simulink model "Actuator_model_discrete"  (R2015b)
settings: Solver=FixedStepAuto  StartTime=0.0  StopTime=50  FixedStep=0.004  RelTol=1e-3
values from neighbouring files (symbols this model uses):
  Bv = 10 / ((180/pi) * 1000)    (= 0.000174532925199)    [initialize_param_mdeg.m]    (also in intialize_param.m = 8)
  Jeq = 0.2740    (= 0.274)    [initialize_param_mdeg.m]    (also in intialize_param.m)
  Km = 0.0429    [initialize_param_mdeg.m]    (also in intialize_param.m)
  Kp = wn / (2*zeta)    (= 4297183.46348)    [initialize_param_mdeg.m]    (also in intialize_param.m = 50)
  Kr = 160    [initialize_param_mdeg.m]    (also in intialize_param.m)
  Kv = wn^2 * Bv / (Kp*Kr*Km)    (= 437.062937063)    [initialize_param_mdeg.m]    (also in intialize_param.m = 233.1002331)
  Tv = (Jeq/Bv)    (= 1569.90435866)    [initialize_param_mdeg.m]    (also in intialize_param.m = 0.03425)
settings Model: Creator=mohit  LastModifiedBy=mohit
settings SolverCC: ZeroCrossControl=DisableAll

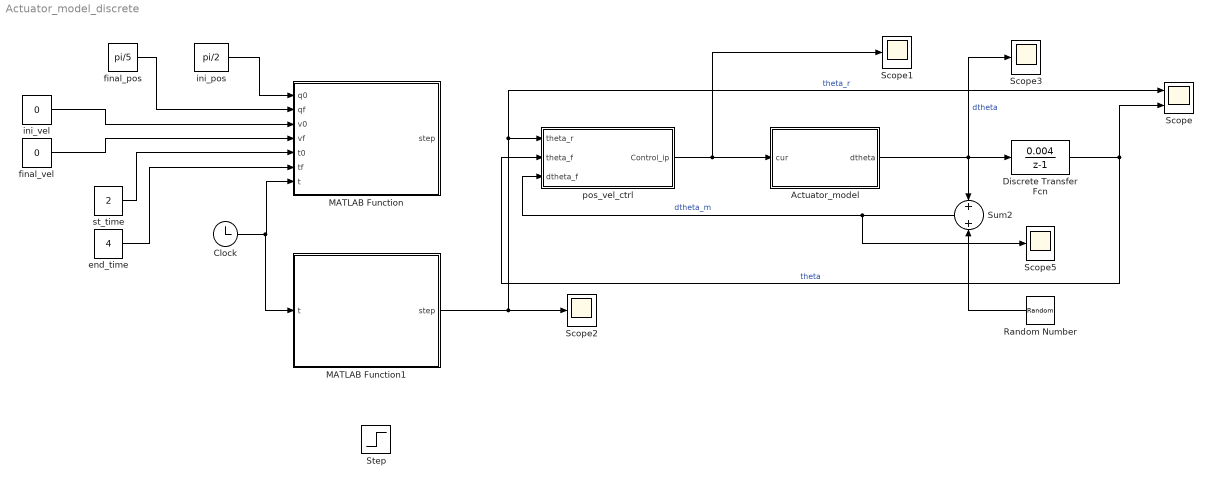
== system Actuator_model_discrete ==
  Actuator_model : Subsystem
  Clock : Clock
  Discrete Transfer Fcn : DiscreteTransferFcn  Numerator=[0.004]  Denominator=[1 -1]
  MATLAB Function : MATLAB Function  TreatAsAtomicUnit=on
  MATLAB Function1 : MATLAB Function  TreatAsAtomicUnit=on
  Random Number : RandomNumber  Variance=0.001 * (pi / 180) * 1000  SampleTime=0.004
  Scope : Scope  NumInputPorts=2
  Scope{1..3,5} (4 alike) : Scope
  Step : Step  Time=4  After=pi/2  SampleTime=0.004
  Sum2 : Sum
  end_time : Constant  Value=4
  final_pos : Constant  Value=pi/5
  final_vel : Constant  Value=0
  ini_pos : Constant  Value=pi/2
  ini_vel : Constant  Value=0
  pos_vel_ctrl : Subsystem
  st_time : Constant  Value=2
  wires:
  Discrete Transfer Fcn/1 -> Scope/2, pos_vel_ctrl/2(theta_f)  "theta"
  Actuator_model/1(dtheta) -> Scope3/1, Discrete Transfer Fcn/1, Sum2/1  "dtheta"
  Sum2/1 -> pos_vel_ctrl/3(dtheta_f), Scope5/1  "dtheta_m"
  Clock/1 -> MATLAB Function1/1(t), MATLAB Function/7(t)
  ini_pos/1 -> MATLAB Function/1(q0)
  final_pos/1 -> MATLAB Function/2(qf)
  ini_vel/1 -> MATLAB Function/3(v0)
  final_vel/1 -> MATLAB Function/4(vf)
  st_time/1 -> MATLAB Function/5(t0)
  end_time/1 -> MATLAB Function/6(tf)
  Random Number/1 -> Sum2/2
  pos_vel_ctrl/1(Control_ip) -> Scope1/1, Actuator_model/1(cur)
  MATLAB Function1/1(step) -> Scope/1, pos_vel_ctrl/1(theta_r), Scope2/1  "theta_r"

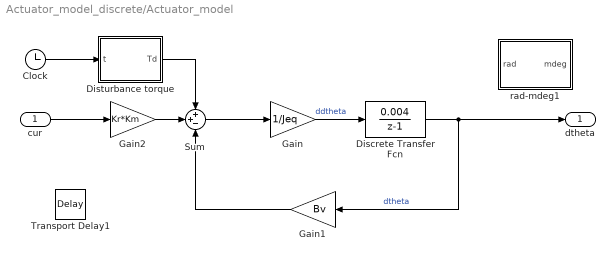
== system Actuator_model_discrete/Actuator_model ==
  cur : Inport
  Clock : Clock
  Discrete Transfer Fcn : DiscreteTransferFcn  Numerator=[0.004]  Denominator=[1 -1]
  Disturbance torque : MATLAB Function  TreatAsAtomicUnit=on
  Gain : Gain  Gain=1/Jeq
  Gain1 : Gain  Gain=Bv
  Gain2 : Gain  Gain=Kr*Km
  Sum : Sum  Inputs=++-
  Transport Delay1 : TransportDelay  DelayTime=0.004
  rad-mdeg1 : MATLAB Function  TreatAsAtomicUnit=on
  dtheta : Outport
  wires:
  Gain2/1 -> Sum/2
  Sum/1 -> Gain/1
  Gain1/1 -> Sum/3
  Gain/1 -> Discrete Transfer Fcn/1  "ddtheta"
  Clock/1 -> Disturbance torque/1(t)
  Disturbance torque/1(Td) -> Sum/1
  cur/1 -> Gain2/1
  Discrete Transfer Fcn/1 -> dtheta/1, Gain1/1  "dtheta"

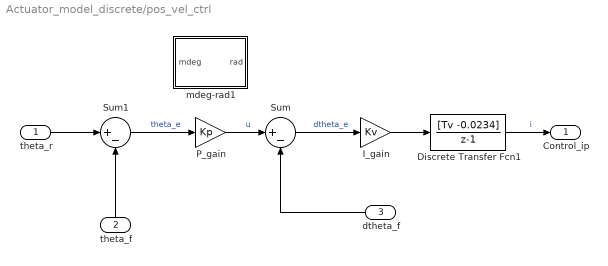
== system Actuator_model_discrete/pos_vel_ctrl ==
  theta_r : Inport
  theta_f : Inport  Port=2
  dtheta_f : Inport  Port=3
  Discrete Transfer Fcn1 : DiscreteTransferFcn  Numerator=[Tv -0.0234]  Denominator=[1 -1]
  I_gain : Gain  Gain=Kv
  P_gain : Gain  Gain=Kp
  Sum : Sum  Inputs=|+-
  Sum1 : Sum  Inputs=|+-
  mdeg-rad1 : MATLAB Function  TreatAsAtomicUnit=on
  Control_ip : Outport
  wires:
  theta_r/1 -> Sum1/1
  dtheta_f/1 -> Sum/2
  theta_f/1 -> Sum1/2
  Discrete Transfer Fcn1/1 -> Control_ip/1  "i"
  Sum/1 -> I_gain/1  "dtheta_e"
  Sum1/1 -> P_gain/1  "theta_e"
  P_gain/1 -> Sum/1  "u"
  I_gain/1 -> Discrete Transfer Fcn1/1

== matlab function Actuator_model_discrete/MATLAB Function ==
  settings: updateMethod=DISCRETE  sampleTime=0.004
  data: q0 input; qf input; v0 input; vf input; t0 input; tf input; t input; step output
function step = smoothstep(q0,qf,v0,vf,t0,tf,t)
    Q = [q0 v0 qf vf]';
    T = zeros(4); A = zeros(4,1);
    ti = 0;
    tn = tf-t0;
    T = [1 ti ti^2  ti^3; ...
         0  1  2*ti 3*ti^2; ...
         1 tn tn^2  tn^3; ...
         0  1  2*tn 3*tn^2];
    A = T \ Q;

    if t <= t0
        step = q0;

    elseif t > t0 && t <= tf
        step = A(4)*((t-t0)^3) + A(3)*((t-t0)^2) + A(2)*(t-t0) + A(1);
    
    else
        step = qf;
    end
end

== matlab function Actuator_model_discrete/Actuator_model/Disturbance torque ==
  settings: updateMethod=DISCRETE  sampleTime=0.004
  data: Td output; t input
function Td = gen_dist(t)
%#codegen

% t = 0:0.004:20
if t > 5 & t < 10
    Td = -1;
else
    Td = 0;
end
end

== matlab function Actuator_model_discrete/pos_vel_ctrl/mdeg-rad1 ==
  data: rad output; mdeg input
function rad = mDegToRad(mdeg)
%#codegen

rad = mdeg / ((pi/180) * 1000);

== matlab function Actuator_model_discrete/MATLAB Function1 ==
  settings: updateMethod=DISCRETE  sampleTime=0.004
  data: t input; step output
function step = smoothstep(t)
    T = zeros(4); A = zeros(4,1);

    if t < 10
        step = 0;

    elseif t >= 10 && t < 16
        t0 = 10;
        ti = 0;
        tn = 6-ti;
        q0 = 0;
        qf = pi/2;
        v0 = 0; vf = 0;
        Q = [q0 v0 qf vf]';
        T = [1 ti ti^2  ti^3; ...
             0  1  2*ti 3*ti^2; ...
             1 tn tn^2  tn^3; ...
             0  1  2*tn 3*tn^2];
        A = T \ Q;
        step = A(4)*((t-t0)^3) + A(3)*((t-t0)^2) + A(2)*(t-t0) + A(1);
    
    elseif t >= 14 && t < 25
        step = pi/2;

    elseif t >= 25 && t < 28
        t0 = 25;
        ti = 0;
        tn = 3-ti;
        q0 = pi/2;
        qf = pi/4;
        v0 = 0; vf = 0;
        Q = [q0 v0 qf vf]';
        T = [1 ti ti^2  ti^3; ...
             0  1  2*ti 3*ti^2; ...
             1 tn tn^2  tn^3; ...
             0  1  2*tn 3*tn^2];
        A = T \ Q;
        step = A(4)*((t-t0)^3) + A(3)*((t-t0)^2) + A(2)*(t-t0) + A(1);
        
    elseif t >= 28 && t < 35
        step = pi/4;

    elseif t >= 35 && t < 38
        t0 = 35;
        ti = 0;
        tn = 3-ti;
        q0 = pi/4;
        qf = 0;
        v0 = 0; vf = 0;
        Q = [q0 v0 qf vf]';
        T = [1 ti ti^2  ti^3; ...
             0  1  2*ti 3*ti^2; ...
             1 tn tn^2  tn^3; ...
             0  1  2*tn 3*tn^2];
        A = T \ Q;
        step = A(4)*((t-t0)^3) + A(3)*((t-t0)^2) + A(2)*(t-t0) + A(1);
    else
        step = 0;
    end
end

== matlab function Actuator_model_discrete/Actuator_model/rad-mdeg1 ==
  data: rad input; mdeg output
function mdeg = radToMdeg(rad)
%#codegen

mdeg = rad * (pi/180) * 1000;
